simulink model "announcement"  (R2023b)
settings: Solver=VariableStepAuto  StartTime=0.0  StopTime=1.04  RelTol=1e-3
values from neighbouring files (symbols this model uses):
  ka = -2    [announceParameters.m]
  ta = 0.005    [announceParameters.m]
libraries: simulink x3
settings Model: Creator=olavhegg  LastModifiedBy=olavhegg

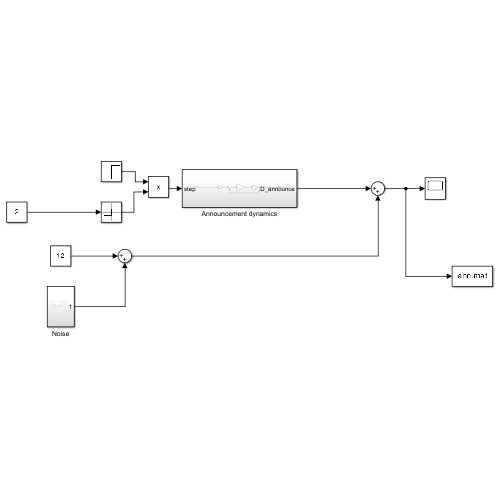
[thumbnail: Simulink's stored preview of the top-level diagram]
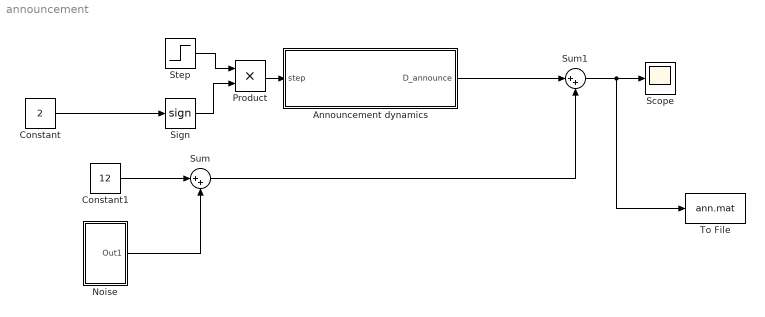
== system announcement ==
  Announcement dynamics : Subsystem
  Constant : Constant  Value=2
  Constant1 : Constant  Value=12
  Noise : Subsystem
  Product : Product
  Scope : Scope
  Sign : Signum
  Step : Step  Time=0.1  SampleTime=0
  Sum : Sum  Inputs=|++
  Sum1 : Sum  Inputs=|++
  To File : ToFile  Filename=ann.mat  MatrixName=anno
  wires:
  Step/1 -> Product/1
  Constant/1 -> Sign/1
  Product/1 -> Announcement dynamics/1(step)
  Sign/1 -> Product/2
  Constant1/1 -> Sum/1
  Noise/1(Out1) -> Sum/2
  Announcement dynamics/1(D_announce) -> Sum1/1
  Sum/1 -> Sum1/2
  Sum1/1 -> To File/1, Scope/1

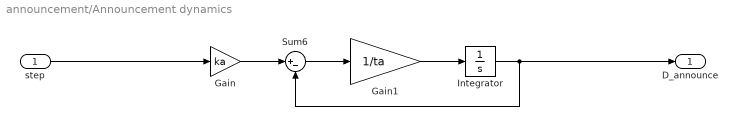
== system announcement/Announcement dynamics ==
  step : Inport
  Gain : Gain  Gain=ka
  Gain1 : Gain  Gain=1/ta
  Integrator : Integrator
  Sum6 : Sum  Inputs=|+-
  D_announce : Outport
  wires:
  Gain/1 -> Sum6/1
  Gain1/1 -> Integrator/1
  Sum6/1 -> Gain1/1
  step/1 -> Gain/1
  Integrator/1 -> D_announce/1, Sum6/2

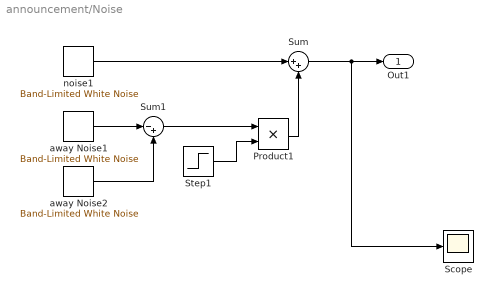
== system announcement/Noise ==
  Product1 : Product
  Scope : Scope
  Step1 : Step  Time=0.12  SampleTime=0
  Sum : Sum  Inputs=|++
  Sum1 : Sum  Inputs=|-+
  away Noise1 : simulink/Sources/Band-Limited White Noise  Cov=[0.000001]  Ts=0.001  seed=[23341]
  away Noise2 : simulink/Sources/Band-Limited White Noise  Cov=[0.0000001]  Ts=0.005  seed=[23342]
  noise1 : simulink/Sources/Band-Limited White Noise  Cov=[0.000001]  Ts=0.001  seed=[23341]
  Out1 : Outport
  wires:
  Product1/1 -> Sum/2
  Step1/1 -> Product1/2
  Sum1/1 -> Product1/1
  Sum/1 -> Scope/1, Out1/1
  noise1/1 -> Sum/1
  away Noise1/1 -> Sum1/1
  away Noise2/1 -> Sum1/2
